simulink model "Induction_Moter_ss_by_19101427"  (R2023b)
settings: Solver=VariableStepAuto  StartTime=0.0  StopTime=10.0  RelTol=1e-3
values from neighbouring files (symbols this model uses):
  J = 3.75    [para.m]
  Lm = 830*10^-6    (= 0.00083)    [para.m]
  Lr = Lm+Llr    (= 0.000848)    [para.m]
  Ls = Lr    (= 0.000848)    [para.m]
  P = 4    [para.m]
  Rr = 0.005724    [para.m]
  Rs = 0.031    [para.m]
undefined symbols (not defined in the file or in its folder): b
settings Model: Creator=jcm52  LastModifiedBy=jcm52

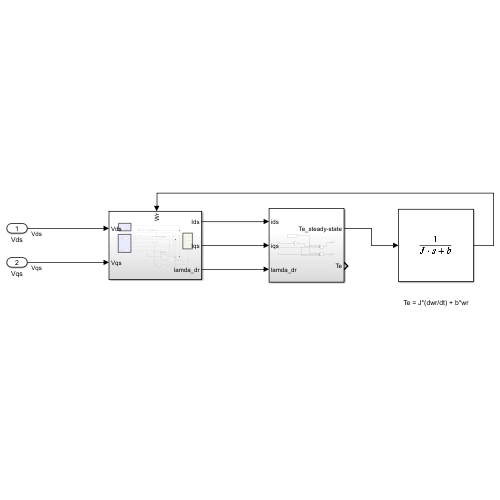
[thumbnail: Simulink's stored preview of the top-level diagram]
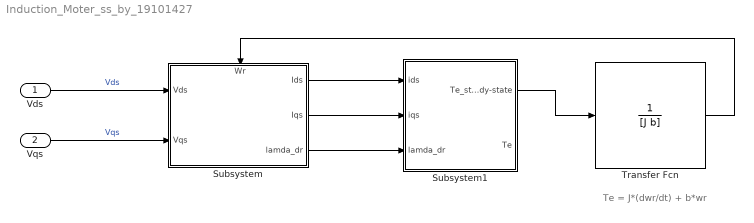
== system Induction_Moter_ss_by_19101427 ==
  note: Te = J*(dwr/dt) + b*wr
  Vds : Inport
  Vqs : Inport  Port=2
  Subsystem : Subsystem
      settings: PortSchema="{\"entries\":[{\"content\":{\"sides\":[{\"content\":{\"connectorIds\":[\"In1\",\"In2\"]},\"type\":\"ConnectorPlacement.EquallySpacedRectSide\",\"uuid\":\"021a9924-daef-431f-9202-fe0cb2092e50\"},{\"content\":{\"connectorIds\":[\"Out1\",\"Out2\",\"Out3\"],\"side\":\"RIGHT\"},\"type\":\"ConnectorPlacement.EquallySpacedRectSide\",\"uuid\":\"d9ecd1b5-b40b-4255-83d5-6b979caeb726\"},{\"content\":{\"connectorIds\":[\"In3\"],\"side\":\"TOP\"},\"type\":\"ConnectorPlacement.EquallySpacedRectSide\",\"uuid\":\"427d6a48-2733-4354-ae42-541a82a28e9a\"}]},\"type\":\"ConnectorPlacement.EquallySpacedConnector\",\"uuid\":\"c06acd2b-8094-49a7-8681-9374d607ed79\"}],\"packageUris\":[\"http://schema.mathworks.com/mf0/Connector/R2020b\"],\"version\":\"1.0\"}"
  Subsystem1 : Subsystem
  Transfer Fcn : TransferFcn  Denominator=[J b]
  wires:
  Subsystem/1(Ids) -> Subsystem1/1(ids)
  Subsystem/2(Iqs) -> Subsystem1/2(iqs)
  Subsystem/3(lamda_dr) -> Subsystem1/3(lamda_dr)
  Transfer Fcn/1 -> Subsystem/3(Wr)
  Vds/1 -> Subsystem/1(Vds)  "Vds"
  Vqs/1 -> Subsystem/2(Vqs)  "Vqs"
  Subsystem1/1(Te_steady-state) -> Transfer Fcn/1

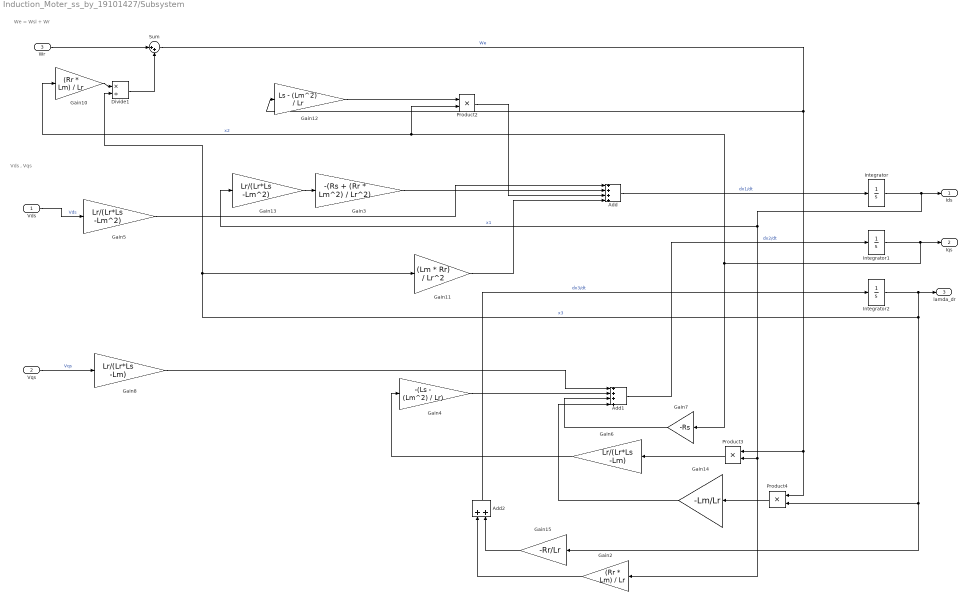
== system Induction_Moter_ss_by_19101427/Subsystem ==
  note: We = Wsl + Wr
  note: Vds , Vqs
  Vds : Inport
  Vqs : Inport  Port=2
  Wr : Inport  Port=3
  Add : Sum  Inputs=++++
  Add1 : Sum  Inputs=++++
  Add2 : Sum
  Divide1 : Product  Inputs=*/
  Gain10 : Gain  Gain=(Rr * Lm) / Lr
  Gain11 : Gain  Gain=(Lm * Rr) / Lr^2
  Gain12 : Gain  Gain=Ls - (Lm^2) / Lr
  Gain13 : Gain  Gain=Lr/(Lr*Ls -Lm^2)
  Gain14 : Gain  Gain=-Lm/Lr
  Gain15 : Gain  Gain=-Rr/Lr
  Gain2 : Gain  Gain=(Rr * Lm) / Lr
  Gain3 : Gain  Gain=-(Rs + (Rr * Lm^2) / Lr^2)
  Gain4 : Gain  Gain=-(Ls - (Lm^2) / Lr)
  Gain5 : Gain  Gain=Lr/(Lr*Ls -Lm^2)
  Gain6 : Gain  Gain=Lr/(Lr*Ls -Lm)
  Gain7 : Gain  Gain=-Rs
  Gain8 : Gain  Gain=Lr/(Lr*Ls -Lm)
  Integrator : Integrator
  Integrator1 : Integrator
  Integrator2 : Integrator
  Product2 : Product
  Product3 : Product
  Product4 : Product
  Sum : Sum  Inputs=|++
  Ids : Outport
  Iqs : Outport  Port=2
  lamda_dr : Outport  Port=3
  wires:
  Integrator1/1 -> Gain10/1, Product2/2, Gain7/1, Iqs/1  "x2"
  Integrator2/1 -> lamda_dr/1, Divide1/2, Gain11/1, Gain15/1, Product4/2  "x3"
  Integrator/1 -> Gain2/1, Product3/2, Gain13/1, Ids/1  "x1"
  Vds/1 -> Gain5/1  "Vds"
  Vqs/1 -> Gain8/1  "Vqs"
  Wr/1 -> Sum/1
  Gain13/1 -> Gain3/1
  Gain3/1 -> Add/2
  Gain10/1 -> Divide1/1
  Divide1/1 -> Sum/2
  Sum/1 -> Product3/1, Product4/1, Gain12/1  "We"
  Gain12/1 -> Product2/1
  Gain5/1 -> Add/1
  Add/1 -> Integrator/1  "dx1/dt"
  Product2/1 -> Add/3
  Gain11/1 -> Add/4
  Gain8/1 -> Add1/1
  Gain4/1 -> Add1/2
  Gain6/1 -> Gain4/1
  Product3/1 -> Gain6/1
  Gain7/1 -> Add1/3
  Product4/1 -> Gain14/1
  Gain14/1 -> Add1/4
  Add1/1 -> Integrator1/1  "dx2/dt"
  Add2/1 -> Integrator2/1  "dx3/dt"
  Gain2/1 -> Add2/1
  Gain15/1 -> Add2/2

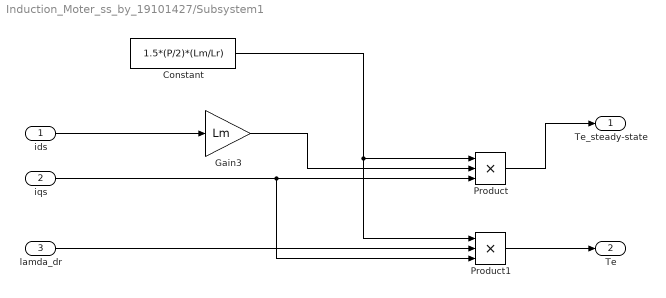
== system Induction_Moter_ss_by_19101427/Subsystem1 ==
  ids : Inport
  iqs : Inport  Port=2
  lamda_dr : Inport  Port=3
  Constant : Constant  Value=1.5*(P/2)*(Lm/Lr)
  Gain3 : Gain  Gain=Lm
  Product : Product  Inputs=3
  Product1 : Product  Inputs=3
  Te_steady-state : Outport
  Te : Outport  Port=2
  wires:
  lamda_dr/1 -> Product1/2
  ids/1 -> Gain3/1
  Product/1 -> Te_steady-state/1
  iqs/1 -> Product1/3, Product/3
  Constant/1 -> Product1/1, Product/1
  Gain3/1 -> Product/2
  Product1/1 -> Te/1
